simulink model "tank_reactor_error_dyn"  (R2018b)
settings: Solver=FixedStepAuto  StartTime=0.0  StopTime=options.T_train  FixedStep=options.dt  RelTol=1e-3
PreLoadFcn:
  | load PIDGainSchedExample.mat
model workspace (MAT data in the model file):
  handle : class17 (value not decoded)
undefined symbols (not defined in the file or in its folder): C, Controllers, D, I, N, options, P, sigbuilder_block
libraries: neural x133, simulink x4
(part 2 of 6)

== system tank_reactor_error_dyn/NN1/Process Output 1 ==
  a : Inport  PortDimensions=1
      mask Display: e = 0.06;c1 = [120 230 180]/255;c2 = ([120 230 180]+0)/(256+128);c3 = ([120 230 180]+128)/(256+128);patch([0 1 1 0],[0 0 1 1],c1);patch([0 1 1 1-e 1-e 0+e],[0 0 1 1-e 0+e 0+e],c2);patch([0 0 1 1-e 0+e 0+e],[0 1 1 1-e 1-e 0+e],c3);plot([0 1 1 0 0],[0 0 1 1 0]);
  mapminmax_reverse : neural/Processing Functions/mapminmax_reverse  xmin=-12958.3118906606632663169875741  xmax=21164.0475047427971730940043926  ymin=-1  ymax=1
  y : Outport  PortDimensions=1
      mask Display: e = 0.06;c1 = [120 230 180]/255;c2 = ([120 230 180]+0)/(256+128);c3 = ([120 230 180]+128)/(256+128);patch([0 1 1 0],[0 0 1 1],c1);patch([0 1 1 1-e 1-e 0+e],[0 0 1 1-e 0+e 0+e],c2);patch([0 0 1 1-e 0+e 0+e],[0 1 1 1-e 1-e 0+e],c3);plot([0 1 1 0 0],[0 0 1 1 0]);
  wires:
  a/1 -> mapminmax_reverse/1
  mapminmax_reverse/1 -> y/1

== system tank_reactor_error_dyn/NN_cex_1/Process Input 1 ==
  x : Inport  PortDimensions=6
      mask Display: e = 0.06;c1 = [120 230 180]/255;c2 = ([120 230 180]+0)/(256+128);c3 = ([120 230 180]+128)/(256+128);patch([0 1 1 0],[0 0 1 1],c1);patch([0 1 1 1-e 1-e 0+e],[0 0 1 1-e 0+e 0+e],c2);patch([0 0 1 1-e 0+e 0+e],[0 1 1 1-e 1-e 0+e],c3);plot([0 1 1 0 0],[0 0 1 1 0]);
  mapminmax : neural/Processing Functions/mapminmax  xmin=[-3.46955594345370688103002976277;-3.46955594345370688103002976277;-3.46955594345370688103002976277;-3.46955594345370688103002976277;-14780.8873093873389734653756022;-14780.8873093873389734653756022]  xmax=[2.91905195298273234527641761815;2.91905195298273234527641761815;2.91905195298273234527641761815;2.91905195298273234527641761815;25176.0648479569572373293340206;25176.0648479569572373293340206]  ymin=-1  ymax=1
  p : Outport  PortDimensions=6
      mask Display: e = 0.06;c1 = [120 230 180]/255;c2 = ([120 230 180]+0)/(256+128);c3 = ([120 230 180]+128)/(256+128);patch([0 1 1 0],[0 0 1 1],c1);patch([0 1 1 1-e 1-e 0+e],[0 0 1 1-e 0+e 0+e],c2);patch([0 0 1 1-e 0+e 0+e],[0 1 1 1-e 1-e 0+e],c3);plot([0 1 1 0 0],[0 0 1 1 0]);
  wires:
  x/1 -> mapminmax/1
  mapminmax/1 -> p/1

== system tank_reactor_error_dyn/NN/Layer 1/Delays 1 ==
  "p{1}" : Inport  PortDimensions=10
      mask Display: e = 0.06;c1 = [120 230 180]/255;c2 = ([120 230 180]+0)/(256+128);c3 = ([120 230 180]+128)/(256+128);patch([0 1 1 0],[0 0 1 1],c1);patch([0 1 1 1-e 1-e 0+e],[0 0 1 1-e 0+e 0+e],c2);patch([0 0 1 1-e 0+e 0+e],[0 1 1 1-e 1-e 0+e],c3);plot([0 1 1 0 0],[0 0 1 1 0]);
  mux : Mux  Inputs=1
      mask Display: e = 0.06;c1 = [120 150 230]/255;c2 = ([120 150 230]+0)/383;c3 = ([120 150 230]+128)/383;patch([0 1 1 0],[0 0 1 1],c1);patch([0 1 1 1-e 1-e 0+e],[0 0 1 1-e 0+e 0+e],c2);patch([0 0 1 1-e 0+e 0+e],[0 1 1 1-e 1-e 0+e],c3);plot([0 1 1 0 0],[0 0 1 1 0]);disp('Mux')
  "pd{1,1}" : Outport
      mask Display: e = 0.06;c1 = [120 230 180]/255;c2 = ([120 230 180]+0)/(256+128);c3 = ([120 230 180]+128)/(256+128);patch([0 1 1 0],[0 0 1 1],c1);patch([0 1 1 1-e 1-e 0+e],[0 0 1 1-e 0+e 0+e],c2);patch([0 0 1 1-e 0+e 0+e],[0 1 1 1-e 1-e 0+e],c3);plot([0 1 1 0 0],[0 0 1 1 0]);
  wires:
  "p{1}"/1 -> mux/1
  mux/1 -> "pd{1,1}"/1

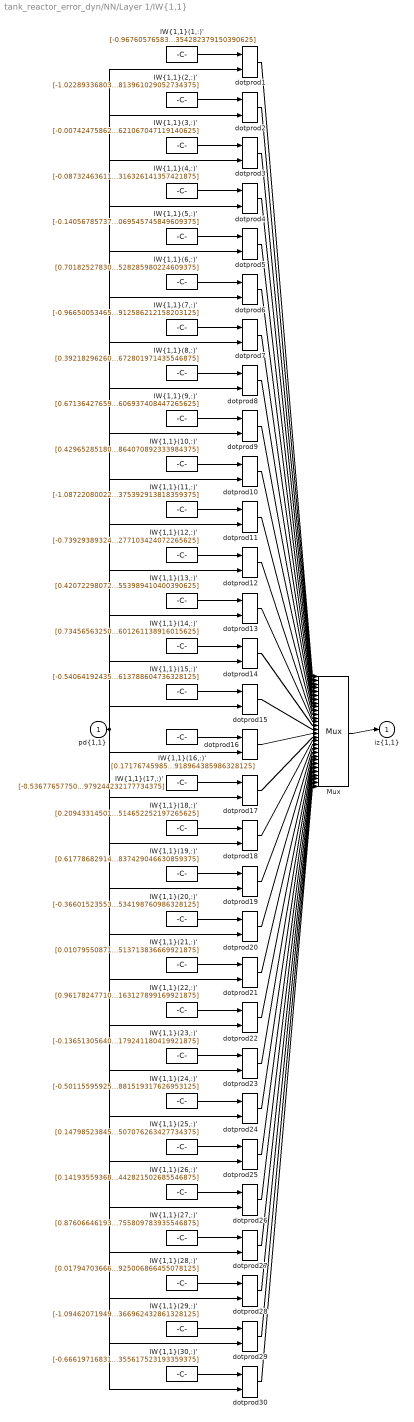
== system tank_reactor_error_dyn/NN/Layer 1/IW{1,1} ==
  "pd{1,1}" : Inport  PortDimensions=10
      mask Display: e = 0.06;c1 = [120 230 180]/255;c2 = ([120 230 180]+0)/(256+128);c3 = ([120 230 180]+128)/(256+128);patch([0 1 1 0],[0 0 1 1],c1);patch([0 1 1 1-e 1-e 0+e],[0 0 1 1-e 0+e 0+e],c2);patch([0 0 1 1-e 0+e 0+e],[0 1 1 1-e 1-e 0+e],c3);plot([0 1 1 0 0],[0 0 1 1 0]);
  "IW{1,1}(1,:)'" : Constant  Value=[-0.96760576583349544588230628505698405206203460693359375;0.8770391079247781274119688532664440572261810302734375;-0.0219785158058380149237454048716244869865477085113525390625;-0.5820181713861958261446716278442181646823883056640625;-0.176131359099816753310818739919341169297695159912109375;0.80717906072376399695400550626800395548343658447265625;0.2250856221299531723101239322204492054879665374755859375;0.373702693428308696521611409480101428925991058349609375;-0.285730596775170209156158307450823485851287841796875;1.111567312552490083277234589331783354282379150390625]
      mask Display: e = 0.06;c1 = [120 150 230]/255;c2 = ([120 150 230]+0)/383;c3 = ([120 150 230]+128)/383;patch([0 1 1 0],[0 0 1 1],c1);patch([0 1 1 1-e 1-e 0+e],[0 0 1 1-e 0+e 0+e],c2);patch([0 0 1 1-e 0+e 0+e],[0 1 1 1-e 1-e 0+e],c3);plot([0 1 1 0 0],[0 0 1 1 0]);disp('Weights');
  "IW{1,1}(10,:)'" : Constant  Value=[0.4296528518094417936623585774214006960391998291015625;-0.217622327924291647516241710036410950124263763427734375;-0.27506649593769993966674292096286080777645111083984375;-0.469924332704204028576810969752841629087924957275390625;-1.050912837992640458395499081234447658061981201171875;0.274270992778577860082833694832515902817249298095703125;0.2954946965743012743388362650875933468341827392578125;-0.19679083633458949176286978399730287492275238037109375;-1.1347591302813186953102331244735978543758392333984375;0.00558595795847411334678067618142449646256864070892333984375]
      mask Display: e = 0.06;c1 = [120 150 230]/255;c2 = ([120 150 230]+0)/383;c3 = ([120 150 230]+128)/383;patch([0 1 1 0],[0 0 1 1],c1);patch([0 1 1 1-e 1-e 0+e],[0 0 1 1-e 0+e 0+e],c2);patch([0 0 1 1-e 0+e 0+e],[0 1 1 1-e 1-e 0+e],c3);plot([0 1 1 0 0],[0 0 1 1 0]);disp('Weights');
  "IW{1,1}(11,:)'" : Constant  Value=[-1.087220800226269989963157058809883892536163330078125;-1.4328123511013910462708054183167405426502227783203125;-0.85972144832092656230315697030164301395416259765625;-0.56462642896457249097608155352645553648471832275390625;-1.49508516079857844971456870553083717823028564453125;0.25839672758254239592901058131246827542781829833984375;-0.38191894340358534254420419529196806252002716064453125;0.270106500234780833036296598947956226766109466552734375;1.0993834340100707702703175527858547866344451904296875;0.9240697255374923368975714765838347375392913818359375]
      mask Display: e = 0.06;c1 = [120 150 230]/255;c2 = ([120 150 230]+0)/383;c3 = ([120 150 230]+128)/383;patch([0 1 1 0],[0 0 1 1],c1);patch([0 1 1 1-e 1-e 0+e],[0 0 1 1-e 0+e 0+e],c2);patch([0 0 1 1-e 0+e 0+e],[0 1 1 1-e 1-e 0+e],c3);plot([0 1 1 0 0],[0 0 1 1 0]);disp('Weights');
  "IW{1,1}(12,:)'" : Constant  Value=[-0.73929389324837890828945319299236871302127838134765625;-0.16974335785768157602859673716011457145214080810546875;0.056792400925659340671369790243261377327144145965576171875;1.3252516622798726775300792724010534584522247314453125;0.7740850330590995920232444404973648488521575927734375;0.12132392786682376362161761562674655579030513763427734375;0.1708054666719572012301142649448593147099018096923828125;0.75632264250021508100729761281399987637996673583984375;-0.419758812120544722024106931712594814598560333251953125;-0.239249287552167066994712740779505111277103424072265625]
      mask Display: e = 0.06;c1 = [120 150 230]/255;c2 = ([120 150 230]+0)/383;c3 = ([120 150 230]+128)/383;patch([0 1 1 0],[0 0 1 1],c1);patch([0 1 1 1-e 1-e 0+e],[0 0 1 1-e 0+e 0+e],c2);patch([0 0 1 1-e 0+e 0+e],[0 1 1 1-e 1-e 0+e],c3);plot([0 1 1 0 0],[0 0 1 1 0]);disp('Weights');
  "IW{1,1}(13,:)'" : Constant  Value=[0.420722980725566297888207145660999231040477752685546875;-0.74009824006719637790041588232270441949367523193359375;-0.8400159086458860446811058864113874733448028564453125;-0.7913045297447605097573841703706420958042144775390625;0.6129681078475466282640127246850170195102691650390625;-0.8596746638172596544080761304940097033977508544921875;0.290461210281355075579767799354158341884613037109375;-0.2694024862551580579150822813971899449825286865234375;0.53539680077279994119265893459669314324855804443359375;-0.9601169906927220498715769281261600553989410400390625]
      mask Display: e = 0.06;c1 = [120 150 230]/255;c2 = ([120 150 230]+0)/383;c3 = ([120 150 230]+128)/383;patch([0 1 1 0],[0 0 1 1],c1);patch([0 1 1 1-e 1-e 0+e],[0 0 1 1-e 0+e 0+e],c2);patch([0 0 1 1-e 0+e 0+e],[0 1 1 1-e 1-e 0+e],c3);plot([0 1 1 0 0],[0 0 1 1 0]);disp('Weights');
  "IW{1,1}(14,:)'" : Constant  Value=[0.7345656325040561540618000435642898082733154296875;-0.42803007769615153410569519110140390694141387939453125;-0.84554514135990810341780843373271636664867401123046875;-0.1047696754001184726856621409751824103295803070068359375;-0.91408144369974431153735849875374697148799896240234375;-0.87714130110913124394045325971092097461223602294921875;0.17009339866629547000087541164248250424861907958984375;0.290309337684379220601016413638717494904994964599609375;0.64897339318505953276172704136115498840808868408203125;-0.371295306470667496601123502841801382601261138916015625]
      mask Display: e = 0.06;c1 = [120 150 230]/255;c2 = ([120 150 230]+0)/383;c3 = ([120 150 230]+128)/383;patch([0 1 1 0],[0 0 1 1],c1);patch([0 1 1 1-e 1-e 0+e],[0 0 1 1-e 0+e 0+e],c2);patch([0 0 1 1-e 0+e 0+e],[0 1 1 1-e 1-e 0+e],c3);plot([0 1 1 0 0],[0 0 1 1 0]);disp('Weights');
  "IW{1,1}(15,:)'" : Constant  Value=[-0.54064192435051439122872807274688966572284698486328125;-0.0335436832600349565947084329309291206300258636474609375;-1.346295502273631594647440579137764871120452880859375;-0.493038271781970849350074104222585447132587432861328125;0.60760741976246179785192680355976335704326629638671875;-0.68146933714951762883771380074904300272464752197265625;1.0983706756652289460163274270598776638507843017578125;-0.04605134032265588428511904339757165871560573577880859375;0.594399662464954570140207579242996871471405029296875;-0.96430593233842387679288776780595071613788604736328125]
      mask Display: e = 0.06;c1 = [120 150 230]/255;c2 = ([120 150 230]+0)/383;c3 = ([120 150 230]+128)/383;patch([0 1 1 0],[0 0 1 1],c1);patch([0 1 1 1-e 1-e 0+e],[0 0 1 1-e 0+e 0+e],c2);patch([0 0 1 1-e 0+e 0+e],[0 1 1 1-e 1-e 0+e],c3);plot([0 1 1 0 0],[0 0 1 1 0]);disp('Weights');
  "IW{1,1}(16,:)'" : Constant  Value=[0.1717674598518805495483974254966597072780132293701171875;-1.8227738936343851339216826090705581009387969970703125;0.81897601940974384948646047632792033255100250244140625;-0.96595167646792867710558994076563976705074310302734375;0.2074597062394892554859637812114669941365718841552734375;1.5411302689041124214242017842479981482028961181640625;-0.404947709113098908151329169413656927645206451416015625;0.3547401202231952321852759268949739634990692138671875;0.34195498187516049082290692240349017083644866943359375;0.03338667600113472133660508234243025071918964385986328125]
      mask Display: e = 0.06;c1 = [120 150 230]/255;c2 = ([120 150 230]+0)/383;c3 = ([120 150 230]+128)/383;patch([0 1 1 0],[0 0 1 1],c1);patch([0 1 1 1-e 1-e 0+e],[0 0 1 1-e 0+e 0+e],c2);patch([0 0 1 1-e 0+e 0+e],[0 1 1 1-e 1-e 0+e],c3);plot([0 1 1 0 0],[0 0 1 1 0]);disp('Weights');
  "IW{1,1}(17,:)'" : Constant  Value=[-0.53677657750629526045571537906653247773647308349609375;0.90230753123584650499111603494384326040744781494140625;0.28843892937913950813566543729393742978572845458984375;0.69914844109946694405977041242294944822788238525390625;0.088083801937797689962650338202365674078464508056640625;-1.0676025926513457164901410578750073909759521484375;-0.4619769138029152788504916316014714539051055908203125;-1.551394658650971702940069008036516606807708740234375;0.25293294392567056139142778192763216793537139892578125;-0.25233058859698809239802130832686088979244232177734375]
      mask Display: e = 0.06;c1 = [120 150 230]/255;c2 = ([120 150 230]+0)/383;c3 = ([120 150 230]+128)/383;patch([0 1 1 0],[0 0 1 1],c1);patch([0 1 1 1-e 1-e 0+e],[0 0 1 1-e 0+e 0+e],c2);patch([0 0 1 1-e 0+e 0+e],[0 1 1 1-e 1-e 0+e],c3);plot([0 1 1 0 0],[0 0 1 1 0]);disp('Weights');
  "IW{1,1}(18,:)'" : Constant  Value=[0.2094331450190706489511427434990764595568180084228515625;0.696379979061731990697126093436963856220245361328125;-1.750098262954347116959752383991144597530364990234375;-0.398905767785253273505219340222538448870182037353515625;-0.538135109363313990371580075589008629322052001953125;-0.350022707822895073892510708901681937277317047119140625;1.52529534185922432953930183430202305316925048828125;-0.24417083370659842245231629931367933750152587890625;1.582116418474436070340516380383633077144622802734375;-1.7687791517987341283202340491698123514652252197265625]
      mask Display: e = 0.06;c1 = [120 150 230]/255;c2 = ([120 150 230]+0)/383;c3 = ([120 150 230]+128)/383;patch([0 1 1 0],[0 0 1 1],c1);patch([0 1 1 1-e 1-e 0+e],[0 0 1 1-e 0+e 0+e],c2);patch([0 0 1 1-e 0+e 0+e],[0 1 1 1-e 1-e 0+e],c3);plot([0 1 1 0 0],[0 0 1 1 0]);disp('Weights');
  "IW{1,1}(19,:)'" : Constant  Value=[0.61778682914916871471433523765881545841693878173828125;0.1465748333359108424023276029402040876448154449462890625;-0.264871921184825775963389560274663381278514862060546875;0.251851456449852462160521326950401999056339263916015625;-0.91608759235413705912520754282013513147830963134765625;0.260152083099477848815439529062132351100444793701171875;-1.4796493035800672988244741645758040249347686767578125;2.059642275254256471583858001395128667354583740234375;-0.370239293019015203167754179958137683570384979248046875;0.45915602702303370818981420597992837429046630859375]
      mask Display: e = 0.06;c1 = [120 150 230]/255;c2 = ([120 150 230]+0)/383;c3 = ([120 150 230]+128)/383;patch([0 1 1 0],[0 0 1 1],c1);patch([0 1 1 1-e 1-e 0+e],[0 0 1 1-e 0+e 0+e],c2);patch([0 0 1 1-e 0+e 0+e],[0 1 1 1-e 1-e 0+e],c3);plot([0 1 1 0 0],[0 0 1 1 0]);disp('Weights');
  "IW{1,1}(2,:)'" : Constant  Value=[-1.0228933680342937595497687652823515236377716064453125;-0.19046509653111975968187152830068953335285186767578125;0.86304655586519507526332972702221013605594635009765625;0.57326276335897663471996565931476652622222900390625;1.45424215784729415901210813899524509906768798828125;0.04860460615202931433653787962612113915383815765380859375;0.568510420914361436217632217449136078357696533203125;-0.7436471332156024960369222753797657787799835205078125;0.462160463711268343356408649924560450017452239990234375;-0.228299472287324556329934921450330875813961029052734375]
      mask Display: e = 0.06;c1 = [120 150 230]/255;c2 = ([120 150 230]+0)/383;c3 = ([120 150 230]+128)/383;patch([0 1 1 0],[0 0 1 1],c1);patch([0 1 1 1-e 1-e 0+e],[0 0 1 1-e 0+e 0+e],c2);patch([0 0 1 1-e 0+e 0+e],[0 1 1 1-e 1-e 0+e],c3);plot([0 1 1 0 0],[0 0 1 1 0]);disp('Weights');
  "IW{1,1}(20,:)'" : Constant  Value=[-0.366015235539588534852128987040487118065357208251953125;-0.88171883663759953453364914821577258408069610595703125;0.40025056294876015794415025084163062274456024169921875;-0.68540340328277549186708483830443583428859710693359375;-0.59544381865096951411686632127384655177593231201171875;-0.85091173049559321039936321540153585374355316162109375;1.09270845367957658567092948942445218563079833984375;-0.137388784200623115250294858924462459981441497802734375;0.767755603158784882822374129318632185459136962890625;0.303989480019571545188483696620096452534198760986328125]
      mask Display: e = 0.06;c1 = [120 150 230]/255;c2 = ([120 150 230]+0)/383;c3 = ([120 150 230]+128)/383;patch([0 1 1 0],[0 0 1 1],c1);patch([0 1 1 1-e 1-e 0+e],[0 0 1 1-e 0+e 0+e],c2);patch([0 0 1 1-e 0+e 0+e],[0 1 1 1-e 1-e 0+e],c3);plot([0 1 1 0 0],[0 0 1 1 0]);disp('Weights');
  "IW{1,1}(21,:)'" : Constant  Value=[0.0107955087137632348148752470251565682701766490936279296875;1.1762465342759049757859202145482413470745086669921875;-0.0613163488384484700599585949021275155246257781982421875;-0.56274155449218898894514495623297989368438720703125;0.555740237947241144667032131110318005084991455078125;-1.400703843194066156030430647660978138446807861328125;0.1256162714214603404183634438595618121325969696044921875;0.371475583213727589271258011649479158222675323486328125;0.734285361009195280956873830291442573070526123046875;-0.26064885020685846228616355801932513713836669921875]
      mask Display: e = 0.06;c1 = [120 150 230]/255;c2 = ([120 150 230]+0)/383;c3 = ([120 150 230]+128)/383;patch([0 1 1 0],[0 0 1 1],c1);patch([0 1 1 1-e 1-e 0+e],[0 0 1 1-e 0+e 0+e],c2);patch([0 0 1 1-e 0+e 0+e],[0 1 1 1-e 1-e 0+e],c3);plot([0 1 1 0 0],[0 0 1 1 0]);disp('Weights');
  "IW{1,1}(22,:)'" : Constant  Value=[0.9617824771093193003679289176943711936473846435546875;0.44064328468005664607431981494300998747348785400390625;0.3286127774954332725343419951968826353549957275390625;0.9193329427419880683913788743666373193264007568359375;1.1925450345544448271795090477098710834980010986328125;0.5717331101020117767319561608019284904003143310546875;-0.508318812790925722566726108198054134845733642578125;0.304763122310873380005347144106053747236728668212890625;-0.364982081123690071944309920581872574985027313232421875;0.92710711811672730231492778329993598163127899169921875]
      mask Display: e = 0.06;c1 = [120 150 230]/255;c2 = ([120 150 230]+0)/383;c3 = ([120 150 230]+128)/383;patch([0 1 1 0],[0 0 1 1],c1);patch([0 1 1 1-e 1-e 0+e],[0 0 1 1-e 0+e 0+e],c2);patch([0 0 1 1-e 0+e 0+e],[0 1 1 1-e 1-e 0+e],c3);plot([0 1 1 0 0],[0 0 1 1 0]);disp('Weights');
  "IW{1,1}(23,:)'" : Constant  Value=[-0.1365130564091787679359413232305087149143218994140625;-1.213465950870285414708860116661526262760162353515625;-0.78532042264329049441329289038549177348613739013671875;-0.0633767506133784686017662579615716822445392608642578125;1.012827498482085974984556742128916084766387939453125;-0.36358149141207862786728810533531941473484039306640625;-1.0519465231777316294170532273710705339908599853515625;-0.486949754469783779864400230508181266486644744873046875;0.293936855628152138297792816956643946468830108642578125;0.14525116302963148040561236484791152179241180419921875]
      mask Display: e = 0.06;c1 = [120 150 230]/255;c2 = ([120 150 230]+0)/383;c3 = ([120 150 230]+128)/383;patch([0 1 1 0],[0 0 1 1],c1);patch([0 1 1 1-e 1-e 0+e],[0 0 1 1-e 0+e 0+e],c2);patch([0 0 1 1-e 0+e 0+e],[0 1 1 1-e 1-e 0+e],c3);plot([0 1 1 0 0],[0 0 1 1 0]);disp('Weights');
  "IW{1,1}(24,:)'" : Constant  Value=[-0.501155959257606919976524295634590089321136474609375;0.792440564103185085542691012960858643054962158203125;-1.713165763562348953286118558025918900966644287109375;0.2139856533101504865168607238956610672175884246826171875;0.8161985977416554849384056069538928568363189697265625;-0.85053942689764483464642808030475862324237823486328125;-0.1669976647801666158610345291890553198754787445068359375;1.362227094580120922984178832848556339740753173828125;1.3787458572366195763692076070583425462245941162109375;-0.7833933982788157113219540406134910881519317626953125]
      mask Display: e = 0.06;c1 = [120 150 230]/255;c2 = ([120 150 230]+0)/383;c3 = ([120 150 230]+128)/383;patch([0 1 1 0],[0 0 1 1],c1);patch([0 1 1 1-e 1-e 0+e],[0 0 1 1-e 0+e 0+e],c2);patch([0 0 1 1-e 0+e 0+e],[0 1 1 1-e 1-e 0+e],c3);plot([0 1 1 0 0],[0 0 1 1 0]);disp('Weights');
  "IW{1,1}(25,:)'" : Constant  Value=[0.14798523845771616169741946578142233192920684814453125;0.8685277138464926327543480510939843952655792236328125;-0.0184293768149740543049741603454094729386270046234130859375;0.0057899676981432619815581830380324390716850757598876953125;-0.312408421129780899949679451310657896101474761962890625;-0.36601725034991117180283026755205355584621429443359375;0.67887311190682797512607749013113789260387420654296875;1.28944638800473310169536489411257207393646240234375;-0.9896485623402460074515829546726308763027191162109375;-0.266025531870186904281894157975330017507076263427734375]
      mask Display: e = 0.06;c1 = [120 150 230]/255;c2 = ([120 150 230]+0)/383;c3 = ([120 150 230]+128)/383;patch([0 1 1 0],[0 0 1 1],c1);patch([0 1 1 1-e 1-e 0+e],[0 0 1 1-e 0+e 0+e],c2);patch([0 0 1 1-e 0+e 0+e],[0 1 1 1-e 1-e 0+e],c3);plot([0 1 1 0 0],[0 0 1 1 0]);disp('Weights');
  "IW{1,1}(26,:)'" : Constant  Value=[0.1419355936893338665516495211704750545322895050048828125;1.4509285175713646509620957658626139163970947265625;0.462861422223198981651393069114419631659984588623046875;0.316800795036313698194163634980213828384876251220703125;0.43736774606802664155935644885175861418247222900390625;0.64432345831802517732711521603050641715526580810546875;-1.1772561285195426439287302855518646538257598876953125;0.78473858100154847416973780127591453492641448974609375;-0.82366254848428843704510882162139751017093658447265625;0.122979370280130506642990440013818442821502685546875]
      mask Display: e = 0.06;c1 = [120 150 230]/255;c2 = ([120 150 230]+0)/383;c3 = ([120 150 230]+128)/383;patch([0 1 1 0],[0 0 1 1],c1);patch([0 1 1 1-e 1-e 0+e],[0 0 1 1-e 0+e 0+e],c2);patch([0 0 1 1-e 0+e 0+e],[0 1 1 1-e 1-e 0+e],c3);plot([0 1 1 0 0],[0 0 1 1 0]);disp('Weights');
  "IW{1,1}(27,:)'" : Constant  Value=[0.87606646193504833508569618061301298439502716064453125;-0.5503439372711227406398393213748931884765625;-0.246573755053914600576803195508546195924282073974609375;-0.385207357636067559969461626678821630775928497314453125;-0.67800739156417855202363398348097689449787139892578125;-0.629552524602530194641758498619310557842254638671875;-0.797952666942423949336671284982003271579742431640625;-0.9413110403176647711376290317275561392307281494140625;0.264474291388262894297866978376987390220165252685546875;0.808036737999269671917090818169526755809783935546875]
      mask Display: e = 0.06;c1 = [120 150 230]/255;c2 = ([120 150 230]+0)/383;c3 = ([120 150 230]+128)/383;patch([0 1 1 0],[0 0 1 1],c1);patch([0 1 1 1-e 1-e 0+e],[0 0 1 1-e 0+e 0+e],c2);patch([0 0 1 1-e 0+e 0+e],[0 1 1 1-e 1-e 0+e],c3);plot([0 1 1 0 0],[0 0 1 1 0]);disp('Weights');
  "IW{1,1}(28,:)'" : Constant  Value=[0.017947036668040095008791467989794909954071044921875;1.739775350476761683893300869385711848735809326171875;-1.026337962663657066286759800277650356292724609375;0.73543640248459940522707256604917347431182861328125;1.469911375899410455048155199619941413402557373046875;-0.69013696085738251984054159038350917398929595947265625;0.89217445192440447687687310462933965027332305908203125;1.384656095532193820218935798038728535175323486328125;0.51691066850944700217240779238636605441570281982421875;-0.49327122262132139240975448046810925006866455078125]
      mask Display: e = 0.06;c1 = [120 150 230]/255;c2 = ([120 150 230]+0)/383;c3 = ([120 150 230]+128)/383;patch([0 1 1 0],[0 0 1 1],c1);patch([0 1 1 1-e 1-e 0+e],[0 0 1 1-e 0+e 0+e],c2);patch([0 0 1 1-e 0+e 0+e],[0 1 1 1-e 1-e 0+e],c3);plot([0 1 1 0 0],[0 0 1 1 0]);disp('Weights');
  "IW{1,1}(29,:)'" : Constant  Value=[-1.0946207194946107055244510775082744657993316650390625;0.6210382469980044728430357281467877328395843505859375;0.1879804631578613494102825143272639252245426177978515625;1.1488585574265599564824924527783878147602081298828125;-0.168956036409220022864730026412871666252613067626953125;-0.2347846605254840512966296728336601518094539642333984375;0.058979017992744887932676789432662189938127994537353515625;0.72044908042839816975089206607663072645664215087890625;-0.097103893282453501711870558210648596286773681640625;0.466473096773016238092424146088887937366962432861328125]
      mask Display: e = 0.06;c1 = [120 150 230]/255;c2 = ([120 150 230]+0)/383;c3 = ([120 150 230]+128)/383;patch([0 1 1 0],[0 0 1 1],c1);patch([0 1 1 1-e 1-e 0+e],[0 0 1 1-e 0+e 0+e],c2);patch([0 0 1 1-e 0+e 0+e],[0 1 1 1-e 1-e 0+e],c3);plot([0 1 1 0 0],[0 0 1 1 0]);disp('Weights');
  "IW{1,1}(3,:)'" : Constant  Value=[-0.007424758620657696296663008439509212621487677097320556640625;-1.3820301983184772876001034092041663825511932373046875;0.87315553362663334002746751139056868851184844970703125;0.2350054958102972546551967525374493561685085296630859375;-0.55047866802660594398588500553159974515438079833984375;0.83237226110455730943016305900528095662593841552734375;-1.101031793721817475528723662137053906917572021484375;-0.39424102033184293958356647635810077190399169921875;-0.382889446768313990165921723018982447683811187744140625;-0.260763084765507857643029865357675589621067047119140625]
      mask Display: e = 0.06;c1 = [120 150 230]/255;c2 = ([120 150 230]+0)/383;c3 = ([120 150 230]+128)/383;patch([0 1 1 0],[0 0 1 1],c1);patch([0 1 1 1-e 1-e 0+e],[0 0 1 1-e 0+e 0+e],c2);patch([0 0 1 1-e 0+e 0+e],[0 1 1 1-e 1-e 0+e],c3);plot([0 1 1 0 0],[0 0 1 1 0]);disp('Weights');
  "IW{1,1}(30,:)'" : Constant  Value=[-0.6661971683182994485861172506702132523059844970703125;-0.6859503636254775660319182861712761223316192626953125;0.75159465293142024844286197549081407487392425537109375;0.82094835814892785919028028729371726512908935546875;0.64301357394976255132945652803755365312099456787109375;-0.821314868144435106245282440795563161373138427734375;-0.302668127514960583201997224023216404020786285400390625;-0.354415793144355284471913591914926655590534210205078125;-0.50629168071408570117597491844207979738712310791015625;0.73326690675042838218899987623444758355617523193359375]
      mask Display: e = 0.06;c1 = [120 150 230]/255;c2 = ([120 150 230]+0)/383;c3 = ([120 150 230]+128)/383;patch([0 1 1 0],[0 0 1 1],c1);patch([0 1 1 1-e 1-e 0+e],[0 0 1 1-e 0+e 0+e],c2);patch([0 0 1 1-e 0+e 0+e],[0 1 1 1-e 1-e 0+e],c3);plot([0 1 1 0 0],[0 0 1 1 0]);disp('Weights');
  "IW{1,1}(4,:)'" : Constant  Value=[-0.08732463611757891597253689042190671898424625396728515625;1.2193960970175805602622176593285985291004180908203125;-0.116887407333546800014545397061738185584545135498046875;-0.103524434890872762959901365320547483861446380615234375;0.8583492311666507390555125311948359012603759765625;-0.320460264922588777825041006508399732410907745361328125;-0.3896090064307047295955044319271109998226165771484375;-0.9837495400719478144679897013702429831027984619140625;0.88675911157954290242599881821661256253719329833984375;-0.31764331922107735817206730644102208316326141357421875]
      mask Display: e = 0.06;c1 = [120 150 230]/255;c2 = ([120 150 230]+0)/383;c3 = ([120 150 230]+128)/383;patch([0 1 1 0],[0 0 1 1],c1);patch([0 1 1 1-e 1-e 0+e],[0 0 1 1-e 0+e 0+e],c2);patch([0 0 1 1-e 0+e 0+e],[0 1 1 1-e 1-e 0+e],c3);plot([0 1 1 0 0],[0 0 1 1 0]);disp('Weights');
  "IW{1,1}(5,:)'" : Constant  Value=[-0.1405678573742802639490179217318654991686344146728515625;1.8769452204440615350478083200869150459766387939453125;-0.9008672652865161722957054735161364078521728515625;-0.68356034985127622771727828876464627683162689208984375;0.4310215467330615890517719890340231359004974365234375;-1.3165481934150868870148087808047421276569366455078125;-0.70540294014327298288691281413775868713855743408203125;0.3699308206567322176994139226735569536685943603515625;0.016169694034388164272098009632827597670257091522216796875;0.08483649716391193640330214975620037876069545745849609375]
      mask Display: e = 0.06;c1 = [120 150 230]/255;c2 = ([120 150 230]+0)/383;c3 = ([120 150 230]+128)/383;patch([0 1 1 0],[0 0 1 1],c1);patch([0 1 1 1-e 1-e 0+e],[0 0 1 1-e 0+e 0+e],c2);patch([0 0 1 1-e 0+e 0+e],[0 1 1 1-e 1-e 0+e],c3);plot([0 1 1 0 0],[0 0 1 1 0]);disp('Weights');
  "IW{1,1}(6,:)'" : Constant  Value=[0.70182527830401875146293377838446758687496185302734375;-0.31533321773393019338271869855816476047039031982421875;-1.3944561320127617509712081300676800310611724853515625;-0.64133378194136347882903237405116669833660125732421875;0.2026225506260409814363043778939754702150821685791015625;-0.192336943841858676318423704287852160632610321044921875;-0.2308758956789348781857285075602703727781772613525390625;-1.7023525465289395253165594112942926585674285888671875;-1.9299395170634310314738968372694216668605804443359375;0.288669990372417861745901745962328277528285980224609375]
      mask Display: e = 0.06;c1 = [120 150 230]/255;c2 = ([120 150 230]+0)/383;c3 = ([120 150 230]+128)/383;patch([0 1 1 0],[0 0 1 1],c1);patch([0 1 1 1-e 1-e 0+e],[0 0 1 1-e 0+e 0+e],c2);patch([0 0 1 1-e 0+e 0+e],[0 1 1 1-e 1-e 0+e],c3);plot([0 1 1 0 0],[0 0 1 1 0]);disp('Weights');
  "IW{1,1}(7,:)'" : Constant  Value=[-0.96650053465591911905363531332113780081272125244140625;0.84776939262057215973555912569281645119190216064453125;0.413880653889037442016984869042062200605869293212890625;0.50623645113457038657855946439667604863643646240234375;-0.995338341442507879008871896076016128063201904296875;0.754977370489878563120100807282142341136932373046875;-0.52548836288382216874737196121714077889919281005859375;-0.53042237966722016739851142119732685387134552001953125;0.31504819032337827433565280443872325122356414794921875;-0.7333687501545977927008834740263409912586212158203125]
      mask Display: e = 0.06;c1 = [120 150 230]/255;c2 = ([120 150 230]+0)/383;c3 = ([120 150 230]+128)/383;patch([0 1 1 0],[0 0 1 1],c1);patch([0 1 1 1-e 1-e 0+e],[0 0 1 1-e 0+e 0+e],c2);patch([0 0 1 1-e 0+e 0+e],[0 1 1 1-e 1-e 0+e],c3);plot([0 1 1 0 0],[0 0 1 1 0]);disp('Weights');
  "IW{1,1}(8,:)'" : Constant  Value=[0.392182962603011997515523034962825477123260498046875;-0.06792833566109778009600717041394091211259365081787109375;0.55573864613154799751981727240490727126598358154296875;-1.02978218570524138186783602577634155750274658203125;0.1324942324138835558766658095919410698115825653076171875;1.6186870552043346460635575567721389234066009521484375;-1.4585394311991339844070125764119438827037811279296875;-0.04676787886599154120403909473679959774017333984375;-0.40699807006023547284456753914128057658672332763671875;-0.415228847256303434942736885204794816672801971435546875]
      mask Display: e = 0.06;c1 = [120 150 230]/255;c2 = ([120 150 230]+0)/383;c3 = ([120 150 230]+128)/383;patch([0 1 1 0],[0 0 1 1],c1);patch([0 1 1 1-e 1-e 0+e],[0 0 1 1-e 0+e 0+e],c2);patch([0 0 1 1-e 0+e 0+e],[0 1 1 1-e 1-e 0+e],c3);plot([0 1 1 0 0],[0 0 1 1 0]);disp('Weights');
  "IW{1,1}(9,:)'" : Constant  Value=[0.671364276593522379954492862452752888202667236328125;0.763598362470879532537537670577876269817352294921875;-0.5634056717374267275744159633177332580089569091796875;-1.3026142240754785550649330616579391062259674072265625;0.0030521537775301068630418033222895246581174433231353759765625;0.104332181965547221569323710355092771351337432861328125;-0.99258955688623407009885113438940607011318206787109375;0.78616527040886696742205685950466431677341461181640625;-0.0599915779508998492364213461769395507872104644775390625;0.167708528573208559553364693783805705606937408447265625]
      mask Display: e = 0.06;c1 = [120 150 230]/255;c2 = ([120 150 230]+0)/383;c3 = ([120 150 230]+128)/383;patch([0 1 1 0],[0 0 1 1],c1);patch([0 1 1 1-e 1-e 0+e],[0 0 1 1-e 0+e 0+e],c2);patch([0 0 1 1-e 0+e 0+e],[0 1 1 1-e 1-e 0+e],c3);plot([0 1 1 0 0],[0 0 1 1 0]);disp('Weights');
  Mux : Mux  Inputs=30
      mask Display: e = 0.06;c1 = [120 150 230]/255;c2 = ([120 150 230]+0)/383;c3 = ([120 150 230]+128)/383;patch([0 1 1 0],[0 0 1 1],c1);patch([0 1 1 1-e 1-e 0+e],[0 0 1 1-e 0+e 0+e],c2);patch([0 0 1 1-e 0+e 0+e],[0 1 1 1-e 1-e 0+e],c3);plot([0 1 1 0 0],[0 0 1 1 0]);disp('Mux');
  dotprod{1..30} (30 alike) : neural/Weight Functions/dotprod
  "iz{1,1}" : Outport
      mask Display: e = 0.06;c1 = [120 230 180]/255;c2 = ([120 230 180]+0)/(256+128);c3 = ([120 230 180]+128)/(256+128);patch([0 1 1 0],[0 0 1 1],c1);patch([0 1 1 1-e 1-e 0+e],[0 0 1 1-e 0+e 0+e],c2);patch([0 0 1 1-e 0+e 0+e],[0 1 1 1-e 1-e 0+e],c3);plot([0 1 1 0 0],[0 0 1 1 0]);
  wires:
  "IW{1,1}(1,:)'"/1 -> dotprod1/1
  "pd{1,1}"/1 -> dotprod1/2, dotprod2/2, dotprod3/2, dotprod4/2, dotprod5/2, dotprod6/2, dotprod7/2, dotprod8/2, dotprod9/2, dotprod10/2, dotprod11/2, dotprod12/2, dotprod13/2, dotprod14/2, dotprod15/2, dotprod16/2, dotprod17/2, dotprod18/2, dotprod19/2, dotprod20/2, dotprod21/2, dotprod22/2, dotprod23/2, dotprod24/2, dotprod25/2, dotprod26/2, dotprod27/2, dotprod28/2, dotprod29/2, dotprod30/2
  dotprod1/1 -> Mux/1
  "IW{1,1}(2,:)'"/1 -> dotprod2/1
  dotprod2/1 -> Mux/2
  "IW{1,1}(3,:)'"/1 -> dotprod3/1
  dotprod3/1 -> Mux/3
  "IW{1,1}(4,:)'"/1 -> dotprod4/1
  dotprod4/1 -> Mux/4
  "IW{1,1}(5,:)'"/1 -> dotprod5/1
  dotprod5/1 -> Mux/5
  "IW{1,1}(6,:)'"/1 -> dotprod6/1
  dotprod6/1 -> Mux/6
  "IW{1,1}(7,:)'"/1 -> dotprod7/1
  dotprod7/1 -> Mux/7
  "IW{1,1}(8,:)'"/1 -> dotprod8/1
  dotprod8/1 -> Mux/8
  "IW{1,1}(9,:)'"/1 -> dotprod9/1
  dotprod9/1 -> Mux/9
  "IW{1,1}(10,:)'"/1 -> dotprod10/1
  dotprod10/1 -> Mux/10
  "IW{1,1}(11,:)'"/1 -> dotprod11/1
  dotprod11/1 -> Mux/11
  "IW{1,1}(12,:)'"/1 -> dotprod12/1
  dotprod12/1 -> Mux/12
  "IW{1,1}(13,:)'"/1 -> dotprod13/1
  dotprod13/1 -> Mux/13
  "IW{1,1}(14,:)'"/1 -> dotprod14/1
  dotprod14/1 -> Mux/14
  "IW{1,1}(15,:)'"/1 -> dotprod15/1
  dotprod15/1 -> Mux/15
  "IW{1,1}(16,:)'"/1 -> dotprod16/1
  dotprod16/1 -> Mux/16
  "IW{1,1}(17,:)'"/1 -> dotprod17/1
  dotprod17/1 -> Mux/17
  "IW{1,1}(18,:)'"/1 -> dotprod18/1
  dotprod18/1 -> Mux/18
  "IW{1,1}(19,:)'"/1 -> dotprod19/1
  dotprod19/1 -> Mux/19
  "IW{1,1}(20,:)'"/1 -> dotprod20/1
  dotprod20/1 -> Mux/20
  "IW{1,1}(21,:)'"/1 -> dotprod21/1
  dotprod21/1 -> Mux/21
  "IW{1,1}(22,:)'"/1 -> dotprod22/1
  dotprod22/1 -> Mux/22
  "IW{1,1}(23,:)'"/1 -> dotprod23/1
  dotprod23/1 -> Mux/23
  "IW{1,1}(24,:)'"/1 -> dotprod24/1
  dotprod24/1 -> Mux/24
  "IW{1,1}(25,:)'"/1 -> dotprod25/1
  dotprod25/1 -> Mux/25
  "IW{1,1}(26,:)'"/1 -> dotprod26/1
  dotprod26/1 -> Mux/26
  "IW{1,1}(27,:)'"/1 -> dotprod27/1
  dotprod27/1 -> Mux/27
  "IW{1,1}(28,:)'"/1 -> dotprod28/1
  dotprod28/1 -> Mux/28
  "IW{1,1}(29,:)'"/1 -> dotprod29/1
  dotprod29/1 -> Mux/29
  "IW{1,1}(30,:)'"/1 -> dotprod30/1
  dotprod30/1 -> Mux/30
  Mux/1 -> "iz{1,1}"/1

== system tank_reactor_error_dyn/NN/Layer 2/Delays 1 ==
  "p{2}" : Inport  PortDimensions=30
      mask Display: e = 0.06;c1 = [120 230 180]/255;c2 = ([120 230 180]+0)/(256+128);c3 = ([120 230 180]+128)/(256+128);patch([0 1 1 0],[0 0 1 1],c1);patch([0 1 1 1-e 1-e 0+e],[0 0 1 1-e 0+e 0+e],c2);patch([0 0 1 1-e 0+e 0+e],[0 1 1 1-e 1-e 0+e],c3);plot([0 1 1 0 0],[0 0 1 1 0]);
  mux : Mux  Inputs=1
      mask Display: e = 0.06;c1 = [120 150 230]/255;c2 = ([120 150 230]+0)/383;c3 = ([120 150 230]+128)/383;patch([0 1 1 0],[0 0 1 1],c1);patch([0 1 1 1-e 1-e 0+e],[0 0 1 1-e 0+e 0+e],c2);patch([0 0 1 1-e 0+e 0+e],[0 1 1 1-e 1-e 0+e],c3);plot([0 1 1 0 0],[0 0 1 1 0]);disp('Mux')
  "pd{2,1}" : Outport
      mask Display: e = 0.06;c1 = [120 230 180]/255;c2 = ([120 230 180]+0)/(256+128);c3 = ([120 230 180]+128)/(256+128);patch([0 1 1 0],[0 0 1 1],c1);patch([0 1 1 1-e 1-e 0+e],[0 0 1 1-e 0+e 0+e],c2);patch([0 0 1 1-e 0+e 0+e],[0 1 1 1-e 1-e 0+e],c3);plot([0 1 1 0 0],[0 0 1 1 0]);
  wires:
  "p{2}"/1 -> mux/1
  mux/1 -> "pd{2,1}"/1
